simulink model "Encoder_reader_simulink"  (R2025a)
settings: Solver=FixedStepAuto  StartTime=0.0  StopTime=inf  FixedStep=0.001  RelTol=1e-3  EnableMultiTasking=on
libraries: stm32f4xxblockslib x3, stm32g4xxblockslib x1
settings Model: STM32="{\"EncoderBlockForG4\":[{\"ID\":\"untitled:1\"},{\"ID\":\"Lab3_Encoder:1\"},{\"ID\":\"Encoder_reader_simulink:1\"}],\"DigitalPortRead\":[{\"ID\":\"Encoder_reader_simulink:20\"},{\"ID\":\"Encoder_reader_simulink:21\"},{\"ID\":\"Encoder_reader_simulink:29\"}]}"  SimulationMode=external  Creator=User  LastModifiedBy=khunb
settings OptimizationCC: DefaultParameterBehavior=Inlined  EnhancedBackFolding=on  PassReuseOutputArgsAs=Individual arguments  ZeroExternalMemoryAtStartup=off  ZeroInternalMemoryAtStartup=off  MaxStackSize=512  OptimizeBlockOrder=speed  DifferentSizesBufferReuse=on  OptimizationCustomize=off  EfficientTunableParamExpr=on
settings DebuggingCC: ParameterTunabilityLossMsg=error
settings HardwareCC: ProdBitPerPointer=32.0  ProdBitPerSizeT=32.0  ProdBitPerPtrDiffT=32.0  ProdLargestAtomicInteger=Long  ProdLargestAtomicFloat=Double  ProdWordSize=32.0  ProdLongLongMode=on  ProdHWDeviceType=ARM Compatible->ARM Cortex-M
settings SFSimCC: MATLABDynamicMemAlloc=off
settings RTWCC: SystemTargetFile=ert.tlc  HardwareBoard=STM32G4xx Based  TemplateMakefile=ert_default_tmf  Toolchain=GNU Tools for ARM Embedded Processors  Description=Embedded Coder
settings CodeAppCC: ForceParamTrailComments=on  IgnoreCustomStorageClasses=off  OperatorAnnotations=on  SimulinkDataObjDesc=on  SFDataObjDesc=on  InsertBlockDesc=on
settings ERTTargetCC: ExtModeTransport=3.0  ExtModeStaticAllocSize=2048.0  TargetLangStandard=C99 (ISO)  CodeReplacementLibrary=ARM Cortex-M  SupportContinuousTime=on

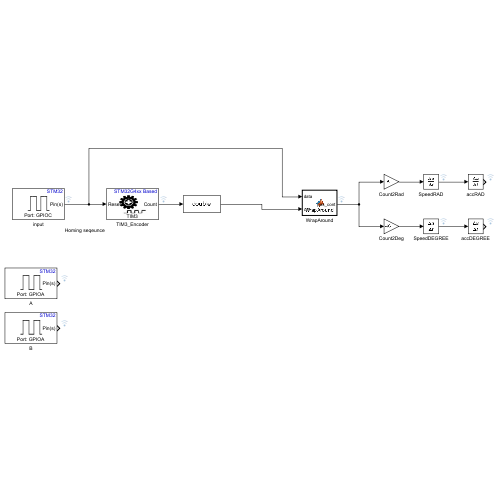
[thumbnail: Simulink's stored preview of the top-level diagram]
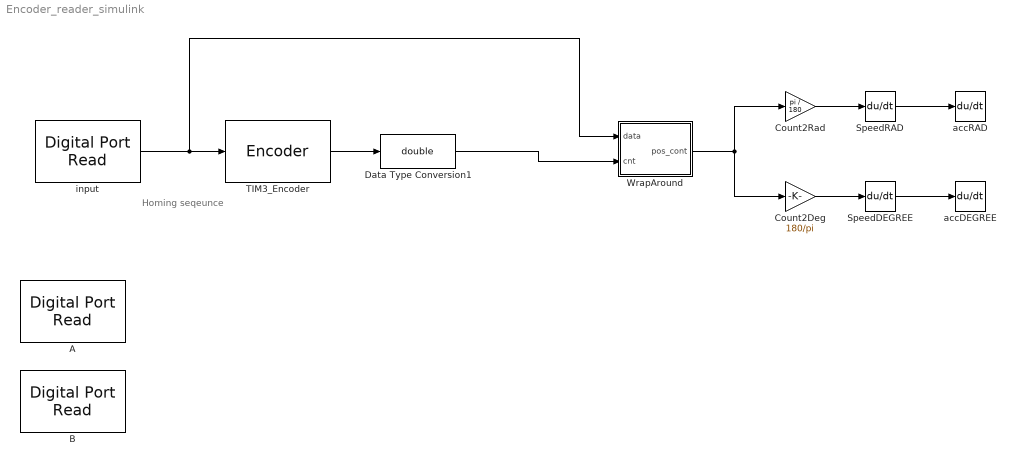
== system Encoder_reader_simulink ==
  note: Homing seqeunce
  A : stm32f4xxblockslib/Digital Port Read  PortName=GPIOA  PinNumber=[6]  ReadOperation=on  IOAsArray=on  SampleTime=-1  EnableSimPort=off  hoistedMaskSrc=ECSoC/ECSimCodegen/Digital Port Read
      settings: LibrarySourceBlock=stm32g4xxblockslib/Digital Port Read
  B : stm32f4xxblockslib/Digital Port Read  PortName=GPIOA  PinNumber=[4]  ReadOperation=on  IOAsArray=on  SampleTime=-1  EnableSimPort=off  hoistedMaskSrc=ECSoC/ECSimCodegen/Digital Port Read
      settings: LibrarySourceBlock=stm32g4xxblockslib/Digital Port Read
  Count2Deg : Gain  Gain=180/pi
  Count2Rad : Gain  Gain=pi / 180
  Data Type Conversion1 : DataTypeConversion  OutDataTypeStr=double  SaturateOnIntegerOverflow=off  RndMeth=Floor
  SpeedDEGREE : Derivative
  SpeedRAD : Derivative
  TIM3_Encoder : stm32g4xxblockslib/Encoder  TimerModule=TIM3  EnableResetInput=on  OutputCountAfterFirstIndex=off  OutputValidIndex=off  OutputDirection=off  OutputStatus=off  SampleTime=-1
  WrapAround : MATLAB Function  TreatAsAtomicUnit=on
  accDEGREE : Derivative
  accRAD : Derivative
  input : stm32f4xxblockslib/Digital Port Read  PortName=GPIOC  PinNumber=[13]  ReadOperation=on  IOAsArray=on  SampleTime=-1  EnableSimPort=off  hoistedMaskSrc=ECSoC/ECSimCodegen/Digital Port Read
      settings: LibrarySourceBlock=stm32g4xxblockslib/Digital Port Read
  wires:
  TIM3_Encoder/1 -> Data Type Conversion1/1
  SpeedRAD/1 -> accRAD/1
  Count2Deg/1 -> SpeedDEGREE/1
  SpeedDEGREE/1 -> accDEGREE/1
  Count2Rad/1 -> SpeedRAD/1
  Data Type Conversion1/1 -> WrapAround/2(cnt)
  input/1 -> WrapAround/1(data), TIM3_Encoder/1
  WrapAround/1(pos_cont) -> Count2Deg/1, Count2Rad/1

== matlab function Encoder_reader_simulink/WrapAround ==
  data: data input; cnt input; pos_cont output
function pos_cont = WrapAround(data,cnt)
persistent last_cnt acc
if isempty(last_cnt)
    last_cnt = int32(cnt);
    acc = int64(0);
end
%homing sequence for wrap around
if data == 1
    last_cnt = int32(0);
    acc = int64(0);
end

MAX_COUNT = int32(61439);
RANGE = int32(MAX_COUNT) + int32(1);   % 61440
HALF = RANGE/2;

delta = int32(cnt) - last_cnt;

% detect wrap
if delta > HALF
    delta = delta - RANGE;   % clockwise large positive -> negative jump (wrap backward)
elseif delta < -HALF
    delta = delta + RANGE;   % counterclockwise large negative -> positive jump (wrap forward)
end

acc = acc + int64(delta);   % accumulate corrected change
pos_cont = double(acc);
last_cnt = int32(cnt);
end
